simulink model "project2old"  (R2012b)
settings: Solver=ode3  StartTime=0.0  StopTime=2  FixedStep=0.01  RelTol=1e-3
values from neighbouring files (symbols this model uses):
  a1 = 500    [RRR_LinkParameters.m]
  a1s = a1*0.001    (= 0.5)    [RRR_LinkParameters.m]
  a2 = 260    [RRR_LinkParameters.m]
  a2s = a2*0.001    (= 0.26)    [RRR_LinkParameters.m]
  a3 = 50    [RRR_LinkParameters.m]
  g = 9.81    [RRR_LinkParameters.m]
  I1 = 0.0123571    [RRR_LinkParameters.m]
  I2 = 0.00189339    [RRR_LinkParameters.m]
  I3 = 0.0000137671    (= 1.37671e-05)    [RRR_LinkParameters.m]
  L1 = 0.246193    [RRR_LinkParameters.m]
  L2 = 0.626297-0.5    (= 0.126297)    [RRR_LinkParameters.m]
  L3 = 0.780098-0.76    (= 0.020098)    [RRR_LinkParameters.m]
  m1 = 0.556965    [RRR_LinkParameters.m]
  m2 = 0.297765    [RRR_LinkParameters.m]
  m3 = 0.0528412    [RRR_LinkParameters.m]
libraries: mblibv1 x23, simulink x8
settings Model: Creator=Sony  LastModifiedBy=Sony
settings SimMechanicsCC: VisDuringSimulation=on
settings ConfigurationSet: Description=SimMechanics 2G

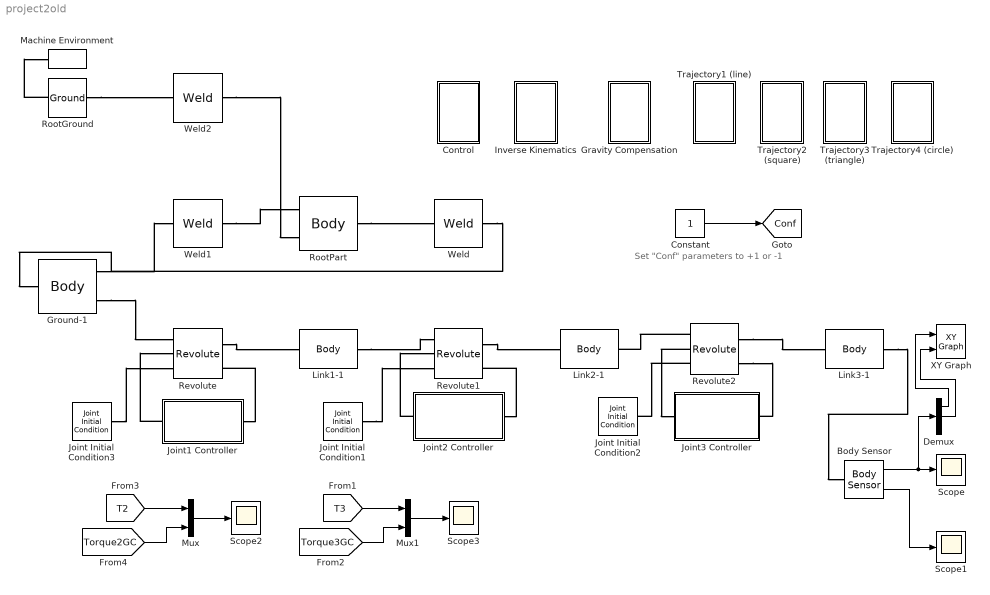
== system project2old ==
  note: Set "Conf" parameters to +1 or -1
  Body Sensor : mblibv1/Sensors &  Actuators/Body Sensor  UpdateFromCAD=off  PhysicalDomain=Mechanical  PortType=blob  Muxed=off  Pose=on  Angle=on  AngleUnits=deg  ArcVelocity=off  ArcVelocityUnits=deg/s  ArcAcceleration=off  ArcAccelerationUnits=deg/s^2  CoordPosition=on  CoordPositionUnits=mm  Velocity=off  VelocityUnits=m/s  Acceleration=off  AccelerationUnits=m/s^2  Quaternion=on  QuaternionDT=off  QuaternionDDT=off  QuaternionUnits=off  OutputVector=[1]  ActiveIO=on  Width=12  DialogClass=MechanicalSensorBlock  ReferenceFrame=Absolute (World)
  Constant : Constant
  Control : Subsystem
  Demux : Demux  Outputs=3
  Gravity Compensation : Subsystem
  Ground-1 : mblibv1/Bodies/Body  LConnTagsString=CS2  RConnTagsString=CS3|CS4  UpdateFromCAD=on  DialogClass=MechanicalBodyBlock  Mass=0.0821588  MassUnits=kg  InertiaUnits=kg*m^2  Inertia=[1.42321e-05,0,0;0,1.42321e-05,0;0,0,2.2987e-05]  Shape=Cylinder  ShapeDims=[1 1]  ShapeUnits=m  ShapeUse=false  Density=1  DensityUnits=kg/m^3  DensityUse=false  GraphicsMode=GFXFILE  GraphicsFileName=Montaj_3R - Ground-1.STL  BodyColorSelMode=COLORPALETTE  BodyColor=[0.894118;0.913725;0.929412]  AttachedToCS=CS1  CG=Right$CG$[0 0 0.01]$WORLD$WORLD$m$[1 0 0;0 1 0;0 0 1]$3x3 Transform$rad$WORLD$false$none  WorkingFrames=Right$CS1$[0 0 0]$WORLD$WORLD$m$[1 0 0;0 1 0;0 0 1]$3x3 Transform$rad$WORLD$false$none#Left$CS2$[0 0 0.01]$WORLD$WORLD$m$[1 0 0;0 1 0;0 0 1]$3x3 Transform$rad$WORLD$true$none#Right$CS3$[0 0 0.01]$WORLD$WORLD$m$[1 0 0;0 1 0;0 0 1]$3x3 Transform$rad$WORLD$true$none#Right$CS4$[0 0 0.02]$WORLD$WORLD$m$[1 0 0;0 1 0;0 0 1]$3x3 Transform$rad$WORLD$true$none  CGPos=[0 0 0.01]  CGRot=[1 0 0;0 1 0;0 0 1]  CS0Pos=[]  CS0Rot=[]  CS1Pos=[0 0 0]  CS1Rot=[1 0 0;0 1 0;0 0 1]  CS2Pos=[0 0 0.01]  CS2Rot=[1 0 0;0 1 0;0 0 1]  CS3Pos=[0 0 0.01]  CS3Rot=[1 0 0;0 1 0;0 0 1]  CS4Pos=[0 0 0.02]  CS4Rot=[1 0 0;0 1 0;0 0 1]  CS5Pos=[]  CS5Rot=[]  CS6Pos=[]  CS6Rot=[]  CS7Pos=[]  CS7Rot=[]  CS8Pos=[]  CS8Rot=[]  CS9Pos=[]  CS9Rot=[]  CS10Pos=[]  CS10Rot=[]  CS11Pos=[]  CS11Rot=[]  CS12Pos=[]  CS12Rot=[]  CS13Pos=[]  CS13Rot=[]  CS14Pos=[]  CS14Rot=[]  CS15Pos=[]  CS15Rot=[]  CS16Pos=[]  CS16Rot=[]  CS17Pos=[]  CS17Rot=[]  CS18Pos=[]  CS18Rot=[]  CS19Pos=[]  CS19Rot=[]  CS20Pos=[]  CS20Rot=[]
  Inverse Kinematics : Subsystem
  Joint Initial Condition1 : mblibv1/Sensors &  Actuators/Joint Initial Condition  UpdateFromCAD=off  LeftPortType=blob  RightPortType=blob  PhysicalDomain=mechanical  DialogClass=InitialConditionBlock  InitialConditions=P1$false$0$m$deg$0$m/s$deg/s#P2$false$0$m$deg$0$m/s$deg/s#P3$false$0$m$deg$0$m/s$deg/s#R1$true$168.86$m$deg$0$m/s$deg/s#R2$false$0$m$deg$0$m/s$deg/s#R3$false$0$m$deg$0$m/s$deg/s#S$false$0$m$deg$0$m/s$deg/s  P1PIC=0  P1VIC=0  P2PIC=0  P2VIC=0  P3PIC=0  P3VIC=0  R1PIC=168.86  R1VIC=0  R2PIC=0  R2VIC=0  R3PIC=0  R3VIC=0  SPIC=0  SVIC=0
  Joint Initial Condition2 : mblibv1/Sensors &  Actuators/Joint Initial Condition  UpdateFromCAD=off  LeftPortType=blob  RightPortType=blob  PhysicalDomain=mechanical  DialogClass=InitialConditionBlock  InitialConditions=P1$false$0$m$deg$0$m/s$deg/s#P2$false$0$m$deg$0$m/s$deg/s#P3$false$0$m$deg$0$m/s$deg/s#R1$true$-104.13$m$deg$0$m/s$deg/s#R2$false$0$m$deg$0$m/s$deg/s#R3$false$0$m$deg$0$m/s$deg/s#S$false$0$m$deg$0$m/s$deg/s  P1PIC=0  P1VIC=0  P2PIC=0  P2VIC=0  P3PIC=0  P3VIC=0  R1PIC=-104.13  R1VIC=0  R2PIC=0  R2VIC=0  R3PIC=0  R3VIC=0  SPIC=0  SVIC=0
  Joint Initial Condition3 : mblibv1/Sensors &  Actuators/Joint Initial Condition  UpdateFromCAD=off  LeftPortType=blob  RightPortType=blob  PhysicalDomain=mechanical  DialogClass=InitialConditionBlock  InitialConditions=P1$false$0$m$deg$0$m/s$deg/s#P2$false$0$m$deg$0$m/s$deg/s#P3$false$0$m$deg$0$m/s$deg/s#R1$true$25.27$m$deg$0$m/s$deg/s#R2$false$0$m$deg$0$m/s$deg/s#R3$false$0$m$deg$0$m/s$deg/s#S$false$0$m$deg$0$m/s$deg/s  P1PIC=0  P1VIC=0  P2PIC=0  P2VIC=0  P3PIC=0  P3VIC=0  R1PIC=25.27  R1VIC=0  R2PIC=0  R2VIC=0  R3PIC=0  R3VIC=0  SPIC=0  SVIC=0
  Joint1 Controller : Subsystem
  Joint2 Controller : Subsystem
  Joint3 Controller : Subsystem
  Link1-1 : mblibv1/Bodies/Body  LConnTagsString=CS2  RConnTagsString=CS3  UpdateFromCAD=on  DialogClass=MechanicalBodyBlock  Mass=0.556965  MassUnits=kg  InertiaUnits=kg*m^2  Inertia=[3.86731e-05,0,-2.08828e-05;0,0.0123589,0;-2.08828e-05,0,0.0123571]  Shape=Cylinder  ShapeDims=[1 1]  ShapeUnits=m  ShapeUse=false  Density=1  DensityUnits=kg/m^3  DensityUse=false  GraphicsMode=GFXFILE  GraphicsFileName=Montaj_3R - Link1-1.STL  BodyColorSelMode=COLORPALETTE  BodyColor=[0.89412 0.91373 0.92941]  AttachedToCS=CS1  CG=Right$CG$[0.246193 0 -0.0098477]$WORLD$WORLD$m$[-1 0 0;0 -1 0;0 0 1]$3x3 Transform$rad$WORLD$false$none  WorkingFrames=Right$CS1$[0.25 0 -0.02]$WORLD$WORLD$m$[-1 0 0;0 -1 0;0 0 1]$3x3 Transform$rad$WORLD$false$none#Left$CS2$[0 0 0.02]$WORLD$WORLD$m$[1 0 0;0 1 0;0 0 1]$3x3 Transform$rad$WORLD$true$none#Right$CS3$[0.5 0 0]$WORLD$WORLD$m$[1 0 0;0 1 0;0 0 1]$3x3 Transform$rad$WORLD$true$none  CGPos=[0.246193 0 -0.0098477]  CGRot=[-1 0 0;0 -1 0;0 0 1]  CS0Pos=[]  CS0Rot=[]  CS1Pos=[0.25 0 -0.02]  CS1Rot=[-1 0 0;0 -1 0;0 0 1]  CS2Pos=[0 0 0.02]  CS2Rot=[1 0 0;0 1 0;0 0 1]  CS3Pos=[0.5 0 0]  CS3Rot=[1 0 0;0 1 0;0 0 1]  CS4Pos=[]  CS4Rot=[]  CS5Pos=[]  CS5Rot=[]  CS6Pos=[]  CS6Rot=[]  CS7Pos=[]  CS7Rot=[]  CS8Pos=[]  CS8Rot=[]  CS9Pos=[]  CS9Rot=[]  CS10Pos=[]  CS10Rot=[]  CS11Pos=[]  CS11Rot=[]  CS12Pos=[]  CS12Rot=[]  CS13Pos=[]  CS13Rot=[]  CS14Pos=[]  CS14Rot=[]  CS15Pos=[]  CS15Rot=[]  CS16Pos=[]  CS16Rot=[]  CS17Pos=[]  CS17Rot=[]  CS18Pos=[]  CS18Rot=[]  CS19Pos=[]  CS19Rot=[]  CS20Pos=[]  CS20Rot=[]
  Link2-1 : mblibv1/Bodies/Body  LConnTagsString=CS2  RConnTagsString=CS3  UpdateFromCAD=on  DialogClass=MechanicalBodyBlock  Mass=0.297765  MassUnits=kg  InertiaUnits=kg*m^2  Inertia=[2.13819e-05,0,-1.07129e-05;0,0.0018952,0;-1.07129e-05,0,0.00189339]  Shape=Cylinder  ShapeDims=[1 1]  ShapeUnits=m  ShapeUse=false  Density=1  DensityUnits=kg/m^3  DensityUse=false  GraphicsMode=GFXFILE  GraphicsFileName=Montaj_3R - Link2-1.STL  BodyColorSelMode=COLORPALETTE  BodyColor=[0.89412 0.91373 0.92941]  AttachedToCS=CS1  CG=Right$CG$[0.626297 0 -0.0297151]$WORLD$WORLD$m$[-1 0 0;0 -1 0;0 0 1]$3x3 Transform$rad$WORLD$false$none  WorkingFrames=Right$CS1$[0.63 0 -0.04]$WORLD$WORLD$m$[-1 0 0;0 -1 0;0 0 1]$3x3 Transform$rad$WORLD$false$none#Left$CS2$[0.5 0 0]$WORLD$WORLD$m$[1 0 0;0 1 0;0 0 1]$3x3 Transform$rad$WORLD$true$none#Right$CS3$[0.76 0 -0.04]$WORLD$WORLD$m$[1 0 0;0 1 0;0 0 1]$3x3 Transform$rad$WORLD$true$none  CGPos=[0.626297 0 -0.0297151]  CGRot=[-1 0 0;0 -1 0;0 0 1]  CS0Pos=[]  CS0Rot=[]  CS1Pos=[0.63 0 -0.04]  CS1Rot=[-1 0 0;0 -1 0;0 0 1]  CS2Pos=[0.5 0 0]  CS2Rot=[1 0 0;0 1 0;0 0 1]  CS3Pos=[0.76 0 -0.04]  CS3Rot=[1 0 0;0 1 0;0 0 1]  CS4Pos=[]  CS4Rot=[]  CS5Pos=[]  CS5Rot=[]  CS6Pos=[]  CS6Rot=[]  CS7Pos=[]  CS7Rot=[]  CS8Pos=[]  CS8Rot=[]  CS9Pos=[]  CS9Rot=[]  CS10Pos=[]  CS10Rot=[]  CS11Pos=[]  CS11Rot=[]  CS12Pos=[]  CS12Rot=[]  CS13Pos=[]  CS13Rot=[]  CS14Pos=[]  CS14Rot=[]  CS15Pos=[]  CS15Rot=[]  CS16Pos=[]  CS16Rot=[]  CS17Pos=[]  CS17Rot=[]  CS18Pos=[]  CS18Rot=[]  CS19Pos=[]  CS19Rot=[]  CS20Pos=[]  CS20Rot=[]
  Link3-1 : mblibv1/Bodies/Body  LConnTagsString=CS2  RConnTagsString=CS1  UpdateFromCAD=on  DialogClass=MechanicalBodyBlock  Mass=0.0528412  MassUnits=kg  InertiaUnits=kg*m^2  Inertia=[3.47692e-06,0,0;0,1.38129e-05,0;0,0,1.37671e-05]  Shape=Cylinder  ShapeDims=[1 1]  ShapeUnits=m  ShapeUse=false  Density=1  DensityUnits=kg/m^3  DensityUse=false  GraphicsMode=GFXFILE  GraphicsFileName=Montaj_3R - Link3-1.STL  BodyColorSelMode=COLORPALETTE  BodyColor=[0.89412 0.91373 0.92941]  AttachedToCS=CS1  CG=Right$CG$[0.780098 0 -0.05]$WORLD$WORLD$m$[1 0 0;0 1 0;0 0 1]$3x3 Transform$rad$WORLD$false$none  WorkingFrames=Right$CS3$[a3 0 0]$Adjoining$Adjoining$mm$[1 0 0;0 1 0;0 0 1]$3x3 Transform$rad$WORLD$false$none#Right$CS1$[0.81 0 -0.06]$WORLD$WORLD$m$[1 0 0;0 1 0;0 0 1]$3x3 Transform$rad$WORLD$true$none#Left$CS2$[0.76 0 -0.04]$WORLD$WORLD$m$[1 0 0;0 1 0;0 0 1]$3x3 Transform$rad$WORLD$true$none  CGPos=[0.780098 0 -0.05]  CGRot=[1 0 0;0 1 0;0 0 1]  CS0Pos=[]  CS0Rot=[]  CS1Pos=[0.81 0 -0.06]  CS1Rot=[1 0 0;0 1 0;0 0 1]  CS2Pos=[0.76 0 -0.04]  CS2Rot=[1 0 0;0 1 0;0 0 1]  CS3Pos=[a3 0 0]  CS3Rot=[1 0 0;0 1 0;0 0 1]  CS4Pos=[]  CS4Rot=[]  CS5Pos=[]  CS5Rot=[]  CS6Pos=[]  CS6Rot=[]  CS7Pos=[]  CS7Rot=[]  CS8Pos=[]  CS8Rot=[]  CS9Pos=[]  CS9Rot=[]  CS10Pos=[]  CS10Rot=[]  CS11Pos=[]  CS11Rot=[]  CS12Pos=[]  CS12Rot=[]  CS13Pos=[]  CS13Rot=[]  CS14Pos=[]  CS14Rot=[]  CS15Pos=[]  CS15Rot=[]  CS16Pos=[]  CS16Rot=[]  CS17Pos=[]  CS17Rot=[]  CS18Pos=[]  CS18Rot=[]  CS19Pos=[]  CS19Rot=[]  CS20Pos=[]  CS20Rot=[]
  Machine Environment : mblibv1/Bodies/Machine Environment  PortType=env  PhysicalDomain=Mechanical  DialogTemplateClass=MECH.MachineEnvironment  SyncWhenCopied=off  Gravity=[0 -9.81 0]  GravityUnits=m/s^2  GravityAsSignal=off  Dimensionality=Auto-detect  AnalysisType=Forward dynamics  LinearAssemblyTolerance=1e-3  LinearAssemblyToleranceUnits=m  AngularAssemblyTolerance=1e-3  AngularAssemblyToleranceUnits=rad  ConstraintSolverType=Stabilizing  ConstraintRelTolerance=1e-4  ConstraintAbsTolerance=1e-4  UseRobustSingularityHandling=off  RedundancyAnalysisToleranceType=Automatically select tolerance  RedundancyAnalysisTolerance=1e-14  StatePerturbationType=Fixed  PerturbationSize=1e-5  VisualizeMachine=on  BodyVisualizationType=Use model default body geometries  BodyColorSelMode=Use model default  DefaultBodyColor=[1 0 0]
  Mux : Mux  Inputs=2
  Mux1 : Mux  Inputs=2
  Revolute : mblibv1/Joints/Revolute  LConnTagsString=__newl0|SA1|SA2  RConnTagsString=__newr0|SA1  UpdateFromCAD=on  NumSAPorts=3  CutJoint=off  MarkAsCut=off  Primitives=prismatic  PrimitiveProps=R1$World$[0,0,1]$revolute  DialogClass=JointBlock  R1Axis=[0,0,1]
  Revolute1 : mblibv1/Joints/Revolute  LConnTagsString=__newl0|SA1|SA2  RConnTagsString=__newr0|SA1  UpdateFromCAD=on  NumSAPorts=3  CutJoint=off  MarkAsCut=off  Primitives=prismatic  PrimitiveProps=R1$World$[0,0,1]$revolute  DialogClass=JointBlock  R1Axis=[0,0,1]
  Revolute2 : mblibv1/Joints/Revolute  LConnTagsString=__newl0|SA1|SA2  RConnTagsString=__newr0|SA1  UpdateFromCAD=on  NumSAPorts=3  CutJoint=off  MarkAsCut=off  Primitives=prismatic  PrimitiveProps=R1$World$[0,0,1]$revolute  DialogClass=JointBlock  R1Axis=[0,0,1]
  RootGround : mblibv1/Bodies/Ground  UpdateFromCAD=on  LeftPortType=env  RightPortType=workingframe  PhysicalDomain=Mechanical  DialogClass=GroundBlock  CoordPosition=[0.368617,0,-0.016321]  CoordPositionUnits=m  StateVectorMgrId=0  MachineId=[1 0]  ShowEnvPort=on
  RootPart : mblibv1/Bodies/Body  LConnTagsString=CS3|CS4  RConnTagsString=CS2  UpdateFromCAD=on  DialogClass=MechanicalBodyBlock  Mass=0  MassUnits=kg  InertiaUnits=kg*m^2  Inertia=[0,0,0;0,0,0;0,0,0]  Shape=Cylinder  ShapeDims=[1 1]  ShapeUnits=m  ShapeUse=false  Density=1  DensityUnits=kg/m^3  DensityUse=false  GraphicsMode=MACHINE_DEFAULT  BodyColorSelMode=MACHINE_DEFAULT  BodyColor=[1;0;0]  AttachedToCS=CS1  CG=Right$CG$[0.368617 0 -0.016321]$WORLD$WORLD$m$[1 0 0;0 1 0;0 0 1]$3x3 Transform$rad$WORLD$false$none  WorkingFrames=Right$CS1$[0 0 0]$WORLD$WORLD$m$[1 0 0;0 1 0;0 0 1]$3x3 Transform$rad$WORLD$false$none#Right$CS2$[0 0 0.01]$WORLD$WORLD$m$[1 0 0;0 1 0;0 0 1]$3x3 Transform$rad$WORLD$true$none#Left$CS3$[0 0 0.01]$WORLD$WORLD$m$[1 0 0;0 1 0;0 0 1]$3x3 Transform$rad$WORLD$true$none#Left$CS4$[0.368617 0 -0.016321]$WORLD$WORLD$m$[1 0 0;0 1 0;0 0 1]$3x3 Transform$rad$WORLD$true$none  CGPos=[0.368617 0 -0.016321]  CGRot=[1 0 0;0 1 0;0 0 1]  CS0Pos=[]  CS0Rot=[]  CS1Pos=[0 0 0]  CS1Rot=[1 0 0;0 1 0;0 0 1]  CS2Pos=[0 0 0.01]  CS2Rot=[1 0 0;0 1 0;0 0 1]  CS3Pos=[0 0 0.01]  CS3Rot=[1 0 0;0 1 0;0 0 1]  CS4Pos=[0.368617 0 -0.016321]  CS4Rot=[1 0 0;0 1 0;0 0 1]  CS5Pos=[]  CS5Rot=[]  CS6Pos=[]  CS6Rot=[]  CS7Pos=[]  CS7Rot=[]  CS8Pos=[]  CS8Rot=[]  CS9Pos=[]  CS9Rot=[]  CS10Pos=[]  CS10Rot=[]  CS11Pos=[]  CS11Rot=[]  CS12Pos=[]  CS12Rot=[]  CS13Pos=[]  CS13Rot=[]  CS14Pos=[]  CS14Rot=[]  CS15Pos=[]  CS15Rot=[]  CS16Pos=[]  CS16Rot=[]  CS17Pos=[]  CS17Rot=[]  CS18Pos=[]  CS18Rot=[]  CS19Pos=[]  CS19Rot=[]  CS20Pos=[]  CS20Rot=[]
  Scope{,1..3} (4 alike) : Scope
      Scope2 settings: YMin=-0.51  YMax=-0.28  SaveName=ScopeData4
      Scope3 settings: TimeRange=2  YMin=-0.011  YMax=0.002  SaveName=ScopeData5
  Trajectory1 (line) : Subsystem
  Trajectory2 (square) : Subsystem
  Trajectory3 (triangle) : Subsystem
  Trajectory4 (circle) : Subsystem
  Weld : mblibv1/Joints/Weld  LConnTagsString=__newl0  RConnTagsString=__newr0  UpdateFromCAD=on  NumSAPorts=0  CutJoint=off  MarkAsCut=off  Primitives=weld  PrimitiveProps=W$WORLD$[0.57735,0.57735,0.57735]$weld  DialogClass=JointBlock  WAxis=[0.57735,0.57735,0.57735]
  Weld1 : mblibv1/Joints/Weld  LConnTagsString=__newl0  RConnTagsString=__newr0  UpdateFromCAD=on  NumSAPorts=0  CutJoint=off  MarkAsCut=off  Primitives=weld  PrimitiveProps=W$WORLD$[0.57735,0.57735,0.57735]$weld  DialogClass=JointBlock  WAxis=[0.57735,0.57735,0.57735]
  Weld2 : mblibv1/Joints/Weld  LConnTagsString=__newl0  RConnTagsString=__newr0  UpdateFromCAD=on  NumSAPorts=0  CutJoint=off  MarkAsCut=off  Primitives=weld  PrimitiveProps=W$WORLD$[0.57735,0.57735,0.57735]$weld  DialogClass=JointBlock  WAxis=[0.57735,0.57735,0.57735]
  XY Graph : simulink/Sinks/XY Graph  xmin=150  xmax=400  ymin=100  ymax=300  st=-1
  tag scope: Conf=global
  wires:
  Body Sensor/1 -> Demux/1, Scope/1
  Body Sensor/2 -> Scope1/1
  Constant/1 -> [Conf]
  Demux/1 -> XY Graph/1
  Demux/2 -> XY Graph/2
  Mux/1 -> Scope2/1
  [T2] -> Mux/1
  [Torque2GC] -> Mux/2
  Mux1/1 -> Scope3/1
  [T3] -> Mux1/1
  [Torque3GC] -> Mux1/2
  connections:
  Revolute1/RConn1 -- Link2-1/LConn1
  Revolute2/LConn1 -- Link2-1/RConn1
  Link1-1/RConn1 -- Revolute1/LConn1
  Link3-1/RConn1 -- Body Sensor/LConn1
  Ground-1/RConn1 -- Weld1/LConn1
  Revolute2/RConn1 -- Link3-1/LConn1
  Weld1/RConn1 -- RootPart/LConn1
  Weld2/RConn1 -- RootPart/LConn2
  Weld/RConn1 -- Ground-1/LConn1
  RootGround/RConn1 -- Weld2/LConn1
  Revolute/RConn1 -- Link1-1/LConn1
  Ground-1/RConn2 -- Revolute/LConn1
  RootPart/RConn1 -- Weld/LConn1
  RootGround/LConn1 -- Machine Environment/RConn1
  Joint2 Controller/LConn1 -- Revolute1/LConn2
  Joint2 Controller/RConn1 -- Revolute1/RConn2
  Revolute2/LConn2 -- Joint3 Controller/LConn1
  Revolute2/RConn2 -- Joint3 Controller/RConn1
  Joint1 Controller/RConn1 -- Revolute/LConn2
  Joint1 Controller/LConn1 -- Revolute/RConn2
  Joint Initial Condition3/RConn1 -- Revolute/LConn3
  Joint Initial Condition1/RConn1 -- Revolute1/LConn3
  Revolute2/LConn3 -- Joint Initial Condition2/RConn1

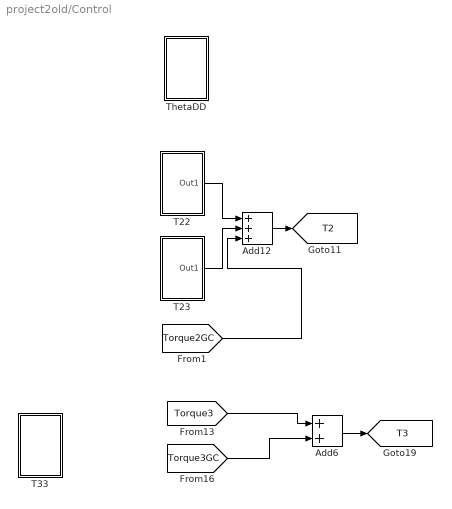
== system project2old/Control ==
  Add12 : Sum  Inputs=+++
  Add6 : Sum
  T22 : Subsystem
  T23 : Subsystem
  T33 : Subsystem
  ThetaDD : Subsystem
  tag scope: T2=global, T3=global
  wires:
  [Torque3] -> Add6/1
  [Torque3GC] -> Add6/2
  Add6/1 -> [T3]
  T22/1(Out1) -> Add12/1
  T23/1(Out1) -> Add12/2
  Add12/1 -> [T2]
  [Torque2GC] -> Add12/3

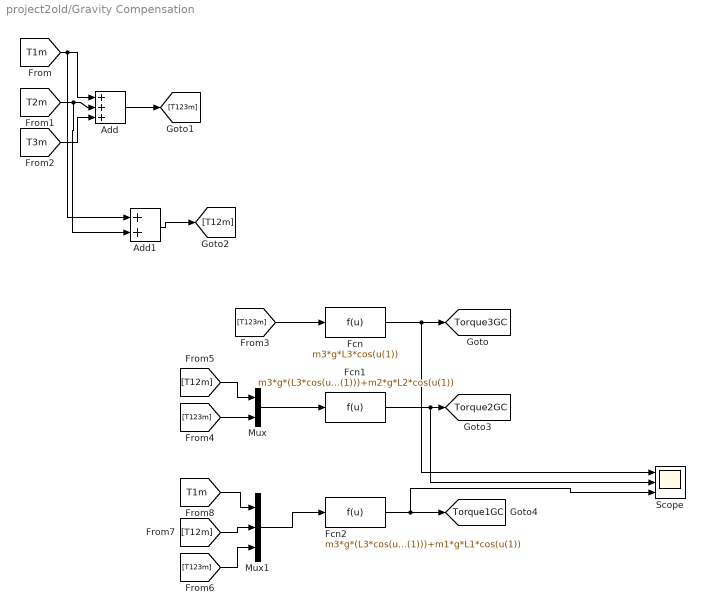
== system project2old/Gravity Compensation ==
  Add : Sum  Inputs=+++
  Add1 : Sum
  Fcn : Fcn  Expr=m3*g*L3*cos(u(1))
  Fcn1 : Fcn  Expr=m3*g*(L3*cos(u(2))+a2s*cos(u(1)))+m2*g*L2*cos(u(1))
  Fcn2 : Fcn  Expr=m3*g*(L3*cos(u(3))+a2s*cos(u(2))+a1s*cos(u(1)))+m2*g*(L2*cos(u(2))+a1s*cos(u(1)))+m1*g*L1*cos(u(1))
  Mux : Mux  Inputs=2
  Mux1 : Mux  Inputs=3
  Scope : Scope  NumInputPorts=3
      settings: YMin=-5~-5~-5  YMax=5~5~5
  tag scope: Torque1GC=global, Torque2GC=global, Torque3GC=global
  wires:
  [T3m] -> Add/3
  [T1m] -> Add1/1, Add/1
  [T2m] -> Add1/2, Add/2
  Add/1 -> [T123m]
  Add1/1 -> [T12m]
  [T123m] -> Fcn/1
  Fcn/1 -> Scope/1, [Torque3GC]
  Fcn1/1 -> Scope/2, [Torque2GC]
  [T12m] -> Mux/1
  [T123m] -> Mux/2
  Mux/1 -> Fcn1/1
  Fcn2/1 -> Scope/3, [Torque1GC]
  Mux1/1 -> Fcn2/1
  [T1m] -> Mux1/1
  [T12m] -> Mux1/2
  [T123m] -> Mux1/3

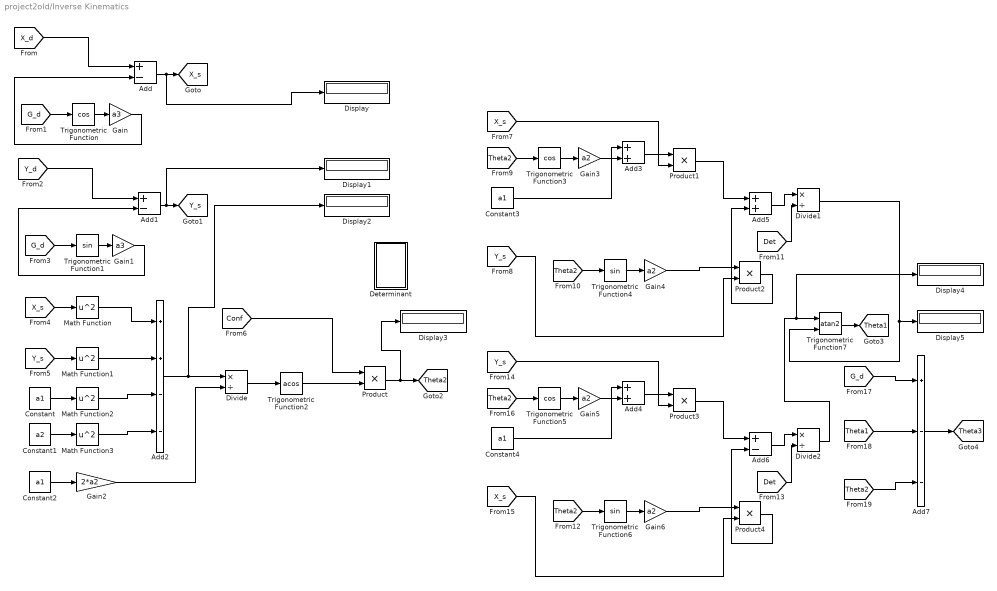
== system project2old/Inverse Kinematics ==
  Add : Sum  Inputs=+-
  Add1 : Sum  Inputs=+-
  Add2 : Sum  Inputs=++--
  Add3 : Sum
  Add4 : Sum
  Add5 : Sum
  Add6 : Sum  Inputs=+-
  Add7 : Sum  Inputs=+--
  Constant{,2..4} (4 alike) : Constant  Value=a1
  Constant1 : Constant  Value=a2
  Determinant : Subsystem
  Display{,1..5} (6 alike) : Display
  Divide : Product  Inputs=*/
  Divide1 : Product  Inputs=*/
  Divide2 : Product  Inputs=*/
  Gain : Gain  Gain=a3
  Gain1 : Gain  Gain=a3
  Gain2 : Gain  Gain=2*a2
  Gain{3..6} (4 alike) : Gain  Gain=a2
  Math Function{,1..3} (4 alike) : Math  Operator=square  SaturateOnIntegerOverflow=on
  Product{,1..4} (5 alike) : Product  RndMeth=Zero
  Trigonometric Function : Trigonometry  Operator=cos
  Trigonometric Function1 : Trigonometry
  Trigonometric Function2 : Trigonometry  Operator=acos
  Trigonometric Function3 : Trigonometry  Operator=cos
  Trigonometric Function4 : Trigonometry
  Trigonometric Function5 : Trigonometry  Operator=cos
  Trigonometric Function6 : Trigonometry
  Trigonometric Function7 : Trigonometry  Operator=atan2
  tag scope: Theta1=global, Theta2=global, Theta3=global, X_s=global, Y_s=global
  wires:
  Add1/1 -> Display1/1, [Y_s]
  [X_d] -> Add/1
  Add/1 -> Display/1, [X_s]
  [Y_d] -> Add1/1
  Gain/1 -> Add/2
  [G_d] -> Trigonometric Function1/1
  Trigonometric Function/1 -> Gain/1
  [G_d] -> Trigonometric Function/1
  Gain1/1 -> Add1/2
  Trigonometric Function1/1 -> Gain1/1
  [X_s] -> Math Function/1
  [Y_s] -> Math Function1/1
  Constant1/1 -> Math Function3/1
  Constant/1 -> Math Function2/1
  Math Function3/1 -> Add2/4
  Math Function2/1 -> Add2/3
  Math Function1/1 -> Add2/2
  Math Function/1 -> Add2/1
  Add2/1 -> Display2/1, Divide/1
  Constant2/1 -> Gain2/1
  Gain2/1 -> Divide/2
  Divide/1 -> Trigonometric Function2/1
  Trigonometric Function2/1 -> Product/2
  [Conf] -> Product/1
  Product/1 -> Display3/1, [Theta2]
  [Theta2] -> Trigonometric Function3/1
  Trigonometric Function3/1 -> Gain3/1
  Gain3/1 -> Add3/2
  Constant3/1 -> Add3/1
  Add3/1 -> Product1/1
  [X_s] -> Product1/2
  [Theta2] -> Trigonometric Function4/1
  Trigonometric Function4/1 -> Gain4/1
  [Y_s] -> Product2/2
  Product2/1 -> Add5/2
  Gain4/1 -> Product2/1
  Add5/1 -> Divide1/1
  [Det] -> Divide1/2
  Product1/1 -> Add5/1
  [Theta2] -> Trigonometric Function5/1
  Trigonometric Function5/1 -> Gain5/1
  Gain5/1 -> Add4/2
  Constant4/1 -> Add4/1
  Add4/1 -> Product3/1
  [Y_s] -> Product3/2
  [Theta2] -> Trigonometric Function6/1
  Trigonometric Function6/1 -> Gain6/1
  [X_s] -> Product4/2
  Product4/1 -> Add6/2
  Gain6/1 -> Product4/1
  Add6/1 -> Divide2/1
  [Det] -> Divide2/2
  Product3/1 -> Add6/1
  Trigonometric Function7/1 -> [Theta1]
  [Theta2] -> Add7/3
  [Theta1] -> Add7/2
  [G_d] -> Add7/1
  Add7/1 -> [Theta3]
  Divide2/1 -> Display4/1, Trigonometric Function7/1
  Divide1/1 -> Display5/1, Trigonometric Function7/2

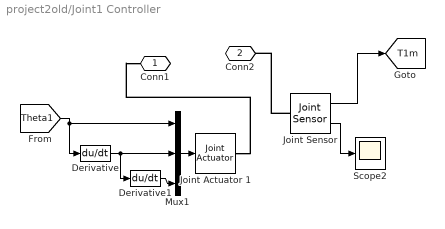
== system project2old/Joint1 Controller ==
  Derivative : Derivative
  Derivative1 : Derivative
  Joint Actuator 1 : mblibv1/Sensors &  Actuators/Joint Actuator  UpdateFromCAD=off  PhysicalDomain=Mechanical  PortType=blob  ActuationStyle=Motion  AngleUnits=rad  ArcVelocityUnits=rad/s  ArcAccelerationUnits=rad/s^2  CoordPositionUnits=m  VelocityUnits=m/s  AccelerationUnits=m/s^2  ForceUnits=N  TorqueUnits=N*m  ActiveIO=on  Width=3  DialogClass=MechanicalActuatorBlock  Primitive=R1  ReferenceFrame=Absolute (World)
  Joint Sensor : mblibv1/Sensors &  Actuators/Joint Sensor  UpdateFromCAD=off  PhysicalDomain=Mechanical  PortType=blob  Muxed=off  Pose=off  Angle=on  AngleUnits=rad  ArcVelocity=off  ArcVelocityUnits=deg/s  ArcAcceleration=off  ArcAccelerationUnits=deg/s^2  CoordPosition=on  CoordPositionUnits=m  Velocity=off  VelocityUnits=m/s  Acceleration=off  AccelerationUnits=m/s^2  Quaternion=on  QuaternionDT=off  QuaternionDDT=off  QuaternionUnits=off  OutputVector=[1]  ActiveIO=on  Width=2  DialogClass=MechanicalSensorBlock  Primitive=R1  Force=off  ForceUnits=N  Torque=on  TorqueUnits=N*m  ReferenceFrame=Absolute (World)  ReactionSensedSide=Base  ReactionReferenceFrame=Absolute (World)  ReactionForce=off  ReactionForceUnits=N  ReactionMoment=off  ReactionMomentUnits=N*m
  Mux1 : Mux  Inputs=3
  Scope2 : Scope
      settings: SaveName=Joint1Torque
  Conn1 : PMIOPort  Port=1  Side=Right
  Conn2 : PMIOPort  Port=2  Side=Left
  tag scope: T1m=global
  wires:
  Mux1/1 -> Joint Actuator 1/1
  Derivative1/1 -> Mux1/3
  Derivative/1 -> Derivative1/1, Mux1/2
  [Theta1] -> Mux1/1, Derivative/1
  Joint Sensor/1 -> [T1m]
  Joint Sensor/2 -> Scope2/1
  connections:
  Joint Sensor/LConn1 -- Conn2/RConn1
  Joint Actuator 1/RConn1 -- Conn1/RConn1

== system project2old/Joint2 Controller ==
  Display : Display
  Joint Actuator : mblibv1/Sensors &  Actuators/Joint Actuator  UpdateFromCAD=off  PhysicalDomain=Mechanical  PortType=blob  ActuationStyle=Force  AngleUnits=deg  ArcVelocityUnits=deg/s  ArcAccelerationUnits=deg/s^2  CoordPositionUnits=m  VelocityUnits=m/s  AccelerationUnits=m/s^2  ForceUnits=N  TorqueUnits=N*m  ActiveIO=on  Width=1  DialogClass=MechanicalActuatorBlock  Primitive=R1  ReferenceFrame=Absolute (World)
  Joint Sensor : mblibv1/Sensors &  Actuators/Joint Sensor  UpdateFromCAD=off  PhysicalDomain=Mechanical  PortType=blob  Muxed=off  Pose=off  Angle=on  AngleUnits=rad  ArcVelocity=off  ArcVelocityUnits=deg/s  ArcAcceleration=off  ArcAccelerationUnits=deg/s^2  CoordPosition=on  CoordPositionUnits=m  Velocity=off  VelocityUnits=m/s  Acceleration=off  AccelerationUnits=m/s^2  Quaternion=on  QuaternionDT=off  QuaternionDDT=off  QuaternionUnits=off  OutputVector=[1]  ActiveIO=on  Width=2  DialogClass=MechanicalSensorBlock  Primitive=R1  Force=off  ForceUnits=N  Torque=on  TorqueUnits=N*m  ReferenceFrame=Absolute (World)  ReactionSensedSide=Base  ReactionReferenceFrame=Absolute (World)  ReactionForce=off  ReactionForceUnits=N  ReactionMoment=off  ReactionMomentUnits=N*m
  Scope2 : Scope
      settings: SaveName=ScopeData3
  Conn1 : PMIOPort  Port=1  Side=Left
  Conn2 : PMIOPort  Port=2  Side=Right
  tag scope: T2m=global
  wires:
  Joint Sensor/1 -> Scope2/1, [T2m]
  Joint Sensor/2 -> Display/1
  [T2] -> Joint Actuator/1
  connections:
  Joint Sensor/LConn1 -- Conn2/RConn1
  Joint Actuator/RConn1 -- Conn1/RConn1

== system project2old/Joint3 Controller ==
  Display : Display
  Joint Actuator : mblibv1/Sensors &  Actuators/Joint Actuator  UpdateFromCAD=off  PhysicalDomain=Mechanical  PortType=blob  ActuationStyle=Force  AngleUnits=rad  ArcVelocityUnits=rad/s  ArcAccelerationUnits=rad/s^2  CoordPositionUnits=m  VelocityUnits=m/s  AccelerationUnits=m/s^2  ForceUnits=N  TorqueUnits=N*m  ActiveIO=on  Width=1  DialogClass=MechanicalActuatorBlock  Primitive=R1  ReferenceFrame=Absolute (World)
  Joint Sensor : mblibv1/Sensors &  Actuators/Joint Sensor  UpdateFromCAD=off  PhysicalDomain=Mechanical  PortType=blob  Muxed=off  Pose=off  Angle=on  AngleUnits=rad  ArcVelocity=off  ArcVelocityUnits=deg/s  ArcAcceleration=off  ArcAccelerationUnits=deg/s^2  CoordPosition=on  CoordPositionUnits=m  Velocity=off  VelocityUnits=m/s  Acceleration=off  AccelerationUnits=m/s^2  Quaternion=on  QuaternionDT=off  QuaternionDDT=off  QuaternionUnits=off  OutputVector=[1]  ActiveIO=on  Width=2  DialogClass=MechanicalSensorBlock  Primitive=R1  Force=off  ForceUnits=N  Torque=on  TorqueUnits=N*m  ReferenceFrame=Absolute (World)  ReactionSensedSide=Base  ReactionReferenceFrame=Absolute (World)  ReactionForce=off  ReactionForceUnits=N  ReactionMoment=off  ReactionMomentUnits=N*m
  Scope2 : Scope
      settings: SaveName=ScopeData2
  Conn1 : PMIOPort  Port=1  Side=Left
  Conn2 : PMIOPort  Port=2  Side=Right
  tag scope: T3m=global
  wires:
  Joint Sensor/1 -> Scope2/1, [T3m]
  [T3] -> Joint Actuator/1
  Joint Sensor/2 -> Display/1
  connections:
  Conn1/RConn1 -- Joint Actuator/RConn1
  Joint Sensor/LConn1 -- Conn2/RConn1

== system project2old/Trajectory1 (line) ==
  Add : Sum
  Constant1 : Constant  Value=pi/2
  Constant2 : Constant  Value=200
  Constant4 : Constant  Value=200
  Integrator : Integrator
  Repeating Sequence : simulink/Sources/Repeating Sequence  rep_seq_t=[0 1 2]  rep_seq_y=[0 100 0]
  tag scope: G_d=global, X_d=global, Y_d=global
  wires:
  Constant4/1 -> Add/1
  Repeating Sequence/1 -> Integrator/1
  Integrator/1 -> Add/2
  Constant2/1 -> [Y_d]
  Add/1 -> [X_d]
  Constant1/1 -> [G_d]

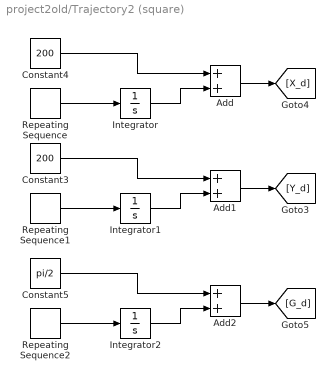
== system project2old/Trajectory2 (square) ==
  Add : Sum
  Add1 : Sum
  Add2 : Sum
  Constant3 : Constant  Value=200
  Constant4 : Constant  Value=200
  Constant5 : Constant  Value=pi/2
  Integrator : Integrator
  Integrator1 : Integrator
  Integrator2 : Integrator
  Repeating Sequence : simulink/Sources/Repeating Sequence  rep_seq_t=[0 1 2 3 4 5 6 7 8 9 10 11 12 13 14]  rep_seq_y=[0 100 0 0 0 0 0 0 0 -100 0 0 0 0 0]
  Repeating Sequence1 : simulink/Sources/Repeating Sequence  rep_seq_t=[0 1 2 3 4 5 6 7 8 9 10 11 12 13 14]  rep_seq_y=[0 0 0 0 0 100 0 0 0 0 0 0 0 -100 0]
  Repeating Sequence2 : simulink/Sources/Repeating Sequence  rep_seq_t=[0 1 2 3 4 5 6 7 8 9 10 11 12 13 14]  rep_seq_y=[0 0 0 pi/2 0 0 0 -pi/2 0 0 0 pi/2 0 0 0]
  wires:
  Add/1 -> [X_d]
  Integrator/1 -> Add/2
  Repeating Sequence/1 -> Integrator/1
  Constant4/1 -> Add/1
  Add1/1 -> [Y_d]
  Integrator1/1 -> Add1/2
  Repeating Sequence1/1 -> Integrator1/1
  Constant3/1 -> Add1/1
  Add2/1 -> [G_d]
  Integrator2/1 -> Add2/2
  Repeating Sequence2/1 -> Integrator2/1
  Constant5/1 -> Add2/1

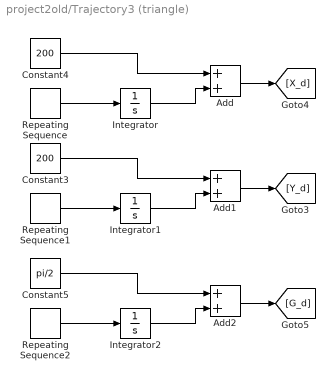
== system project2old/Trajectory3 (triangle) ==
  Add : Sum
  Add1 : Sum
  Add2 : Sum
  Constant3 : Constant  Value=200
  Constant4 : Constant  Value=200
  Constant5 : Constant  Value=pi/2
  Integrator : Integrator
  Integrator1 : Integrator
  Integrator2 : Integrator
  Repeating Sequence : simulink/Sources/Repeating Sequence  rep_seq_t=[0 1 2 3 4 5 6 7 8 9 10]  rep_seq_y=[0 60 0 0 0 -30 0 0 0 -30 0 ]
  Repeating Sequence1 : simulink/Sources/Repeating Sequence  rep_seq_t=[0 1 2 3 4 5 6 7 8 9 10]  rep_seq_y=[0 0 0 0 0 40 0 0 0 -40 0]
  Repeating Sequence2 : simulink/Sources/Repeating Sequence  rep_seq_t=[0 1 2 3 4 5 6 7 8 9 10]  rep_seq_y=[0 0 0 -pi/3.4 0 0 0 pi/2.43 0 0 0]
  wires:
  Add/1 -> [X_d]
  Integrator/1 -> Add/2
  Repeating Sequence/1 -> Integrator/1
  Constant4/1 -> Add/1
  Add1/1 -> [Y_d]
  Integrator1/1 -> Add1/2
  Repeating Sequence1/1 -> Integrator1/1
  Constant3/1 -> Add1/1
  Add2/1 -> [G_d]
  Integrator2/1 -> Add2/2
  Repeating Sequence2/1 -> Integrator2/1
  Constant5/1 -> Add2/1

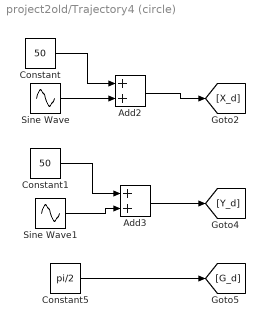
== system project2old/Trajectory4 (circle) ==
  Add2 : Sum
  Add3 : Sum
  Constant : Constant  Value=50
  Constant1 : Constant  Value=50
  Constant5 : Constant  Value=pi/2
  Sine Wave : Sin  Amplitude=20  Frequency=2*pi/100  Phase=pi/2  SampleTime=0
  Sine Wave1 : Sin  Amplitude=20  Frequency=2*pi/100  SampleTime=0
  wires:
  Constant5/1 -> [G_d]
  Constant/1 -> Add2/1
  Sine Wave/1 -> Add2/2
  Constant1/1 -> Add3/1
  Sine Wave1/1 -> Add3/2
  Add2/1 -> [X_d]
  Add3/1 -> [Y_d]

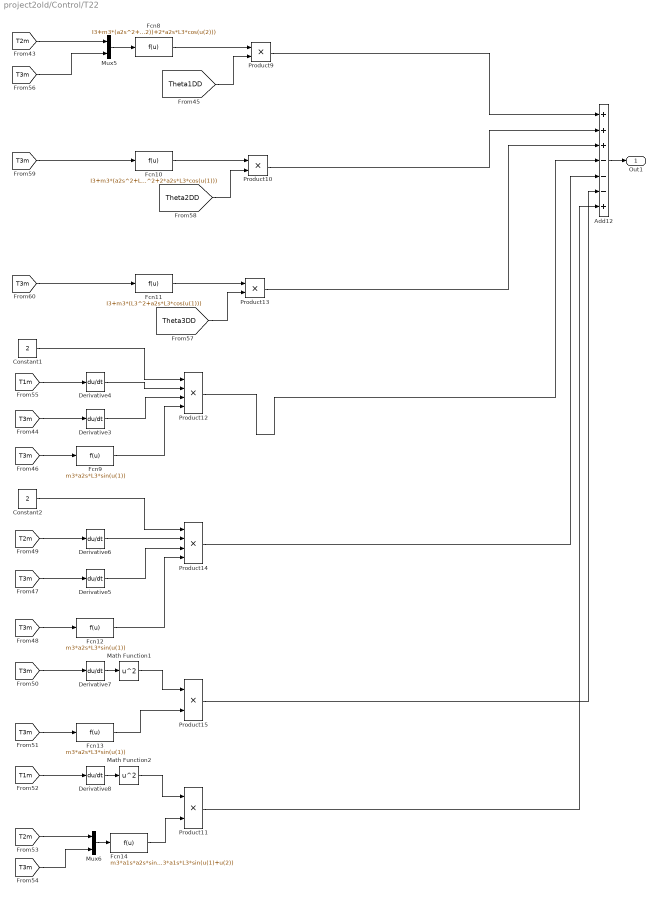
== system project2old/Control/T22 ==
  Add12 : Sum  Inputs=+++---+
  Constant1 : Constant  Value=2
  Constant2 : Constant  Value=2
  Derivative{3..8} (6 alike) : Derivative
  Fcn10 : Fcn  Expr=I3+m3*(a2s^2+L3^2+2*a2s*L3*cos(u(1)))
  Fcn11 : Fcn  Expr=I3+m3*(L3^2+a2s*L3*cos(u(1)))
  Fcn12 : Fcn  Expr=m3*a2s*L3*sin(u(1))
  Fcn13 : Fcn  Expr=m3*a2s*L3*sin(u(1))
  Fcn14 : Fcn  Expr=m3*a1s*a2s*sin(u(1))+m3*a1s*L3*sin(u(1)+u(2))
  Fcn8 : Fcn  Expr=I3+m3*(a2s^2+L3^2+a1s*a2s*cos(u(1))+a1s*L3*cos(u(1)+(2))+2*a2s*L3*cos(u(2)))
  Fcn9 : Fcn  Expr=m3*a2s*L3*sin(u(1))
  Math Function1 : Math  Operator=square  SaturateOnIntegerOverflow=on
  Math Function2 : Math  Operator=square  SaturateOnIntegerOverflow=on
  Mux5 : Mux  Inputs=2
  Mux6 : Mux  Inputs=2
  Product{9..11,13,15} (5 alike) : Product
  Product12 : Product  Inputs=4
  Product14 : Product  Inputs=4
  Out1 : Outport
  wires:
  Add12/1 -> Out1/1
  [T3m] -> Fcn13/1
  [T3m] -> Derivative7/1
  Product10/1 -> Add12/2
  [T3m] -> Fcn10/1
  Fcn9/1 -> Product12/4
  [T1m] -> Derivative4/1
  Math Function2/1 -> Product11/1
  [Theta1DD] -> Product9/2
  [T3m] -> Derivative5/1
  Product11/1 -> Add12/7
  [T3m] -> Fcn12/1
  [Theta2DD] -> Product10/2
  [T3m] -> Fcn9/1
  [T3m] -> Fcn11/1
  Product13/1 -> Add12/3
  Derivative6/1 -> Product14/2
  Product15/1 -> Add12/6
  Product9/1 -> Add12/1
  [T3m] -> Derivative3/1
  Product14/1 -> Add12/5
  [Theta3DD] -> Product13/2
  Derivative8/1 -> Math Function2/1
  [T2m] -> Mux5/1
  Fcn12/1 -> Product14/4
  Constant1/1 -> Product12/1
  Derivative3/1 -> Product12/3
  Derivative7/1 -> Math Function1/1
  Product12/1 -> Add12/4
  [T3m] -> Mux6/2
  Fcn14/1 -> Product11/2
  [T2m] -> Derivative6/1
  Derivative5/1 -> Product14/3
  Fcn11/1 -> Product13/1
  Fcn8/1 -> Product9/1
  Mux6/1 -> Fcn14/1
  Fcn13/1 -> Product15/2
  [T3m] -> Mux5/2
  Mux5/1 -> Fcn8/1
  [T1m] -> Derivative8/1
  Derivative4/1 -> Product12/2
  Fcn10/1 -> Product10/1
  [T2m] -> Mux6/1
  Math Function1/1 -> Product15/1
  Constant2/1 -> Product14/1

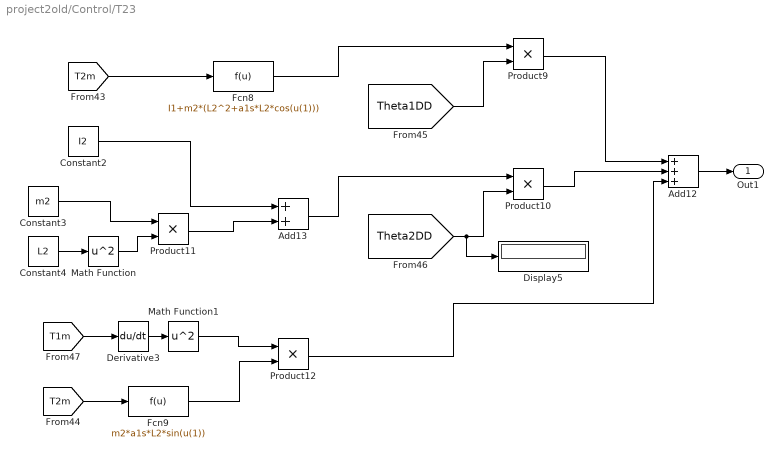
== system project2old/Control/T23 ==
  Add12 : Sum  Inputs=+++
  Add13 : Sum
  Constant2 : Constant  Value=I2
  Constant3 : Constant  Value=m2
  Constant4 : Constant  Value=L2
  Derivative3 : Derivative
  Display5 : Display
  Fcn8 : Fcn  Expr=I1+m2*(L2^2+a1s*L2*cos(u(1)))
  Fcn9 : Fcn  Expr=m2*a1s*L2*sin(u(1))
  Math Function : Math  Operator=square  SaturateOnIntegerOverflow=on
  Math Function1 : Math  Operator=square  SaturateOnIntegerOverflow=on
  Product{9..12} (4 alike) : Product
  Out1 : Outport
  wires:
  [Theta1DD] -> Product9/2
  Product9/1 -> Add12/1
  Math Function1/1 -> Product12/1
  Constant4/1 -> Math Function/1
  Add12/1 -> Out1/1
  [T2m] -> Fcn9/1
  Product11/1 -> Add13/2
  Constant3/1 -> Product11/1
  Math Function/1 -> Product11/2
  Fcn8/1 -> Product9/1
  Derivative3/1 -> Math Function1/1
  Product12/1 -> Add12/3
  [T1m] -> Derivative3/1
  [T2m] -> Fcn8/1
  Constant2/1 -> Add13/1
  Add13/1 -> Product10/1
  Product10/1 -> Add12/2
  [Theta2DD] -> Display5/1, Product10/2
  Fcn9/1 -> Product12/2

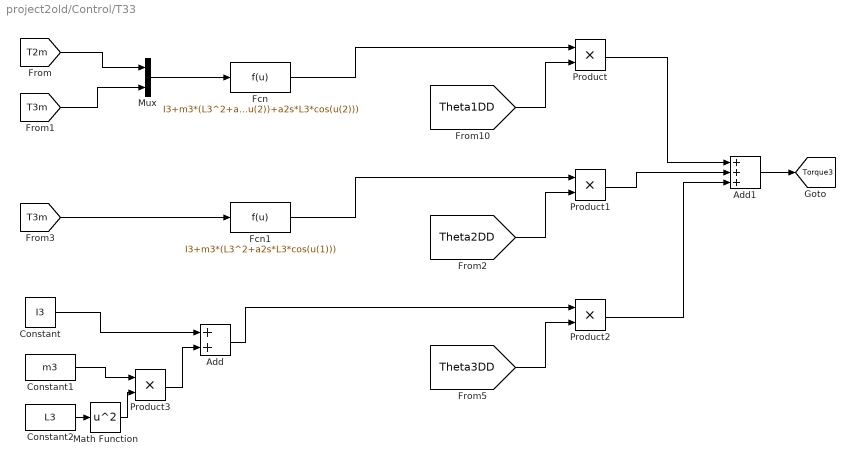
== system project2old/Control/T33 ==
  Add : Sum
  Add1 : Sum  Inputs=+++
  Constant : Constant  Value=I3
  Constant1 : Constant  Value=m3
  Constant2 : Constant  Value=L3
  Fcn : Fcn  Expr=I3+m3*(L3^2+a1s*L3*cos(u(1)+u(2))+a2s*L3*cos(u(2)))
  Fcn1 : Fcn  Expr=I3+m3*(L3^2+a2s*L3*cos(u(1)))
  Math Function : Math  Operator=square  SaturateOnIntegerOverflow=on
  Mux : Mux  Inputs=2
  Product{,1..3} (4 alike) : Product
  tag scope: Torque3=global
  wires:
  Mux/1 -> Fcn/1
  [T3m] -> Fcn1/1
  Constant/1 -> Add/1
  [T2m] -> Mux/1
  [T3m] -> Mux/2
  Fcn1/1 -> Product1/1
  [Theta2DD] -> Product1/2
  Product1/1 -> Add1/2
  Product2/1 -> Add1/3
  Product/1 -> Add1/1
  Fcn/1 -> Product/1
  Add/1 -> Product2/1
  [Theta3DD] -> Product2/2
  [Theta1DD] -> Product/2
  Constant2/1 -> Math Function/1
  Math Function/1 -> Product3/2
  Constant1/1 -> Product3/1
  Product3/1 -> Add/2
  Add1/1 -> [Torque3]

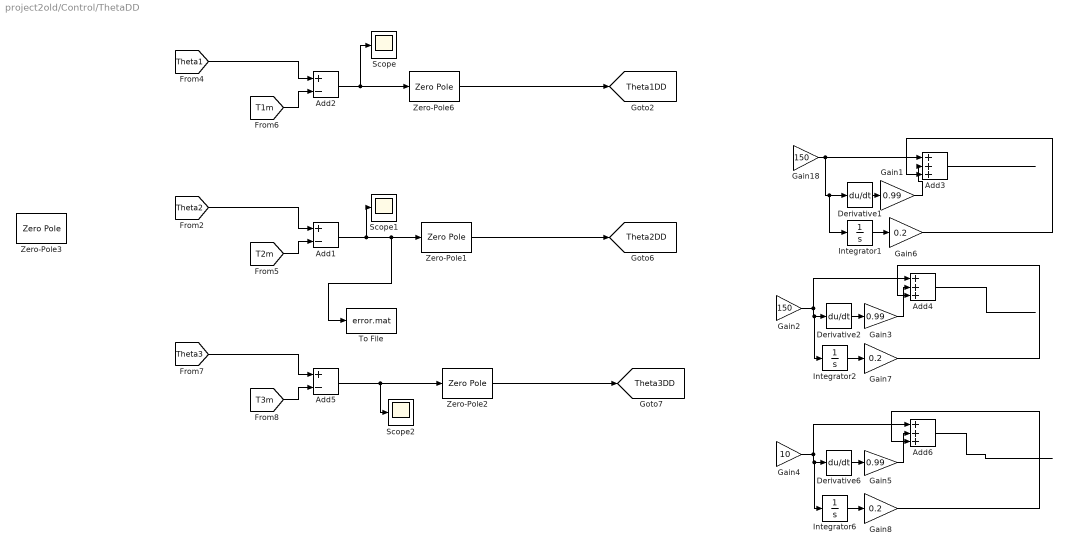
== system project2old/Control/ThetaDD ==
  Add1 : Sum  Inputs=+-
  Add2 : Sum  Inputs=+-
  Add3 : Sum  Inputs=+++
  Add4 : Sum  Inputs=+++
  Add5 : Sum  Inputs=+-
  Add6 : Sum  Inputs=+++
  Derivative1 : Derivative
  Derivative2 : Derivative
  Derivative6 : Derivative
  Gain1 : Gain  Gain=0.99
  Gain18 : Gain  Gain=150
  Gain2 : Gain  Gain=150
  Gain3 : Gain  Gain=0.99
  Gain4 : Gain  Gain=10
  Gain5 : Gain  Gain=0.99
  Gain6 : Gain  Gain=0.2
  Gain7 : Gain  Gain=0.2
  Gain8 : Gain  Gain=0.2
  Integrator1 : Integrator
  Integrator2 : Integrator
  Integrator6 : Integrator
  Scope : Scope
      settings: SaveName=ScopeData7
  Scope1 : Scope
      settings: YMin=-0.09  YMax=0.06  SaveName=ScopeData8
  Scope2 : Scope
      settings: YMin=-1.75  YMax=0.75  SaveName=ScopeData9
  To File : ToFile  Filename=error.mat  MatrixName=error
  Zero-Pole1 : ZeroPole  Zeros=[-10]  Poles=[-20]  Gain=[10000]
  Zero-Pole2 : ZeroPole  Zeros=[-10]  Poles=[-20]  Gain=[10000]
  Zero-Pole3 : ZeroPole  Zeros=[-0.01]  Poles=[-0.009]  Gain=[10000]
  Zero-Pole6 : ZeroPole  Zeros=[-10]  Poles=[-20]  Gain=[10000]
  tag scope: Theta1DD=global, Theta2DD=global, Theta3DD=global
  wires:
  [T2m] -> Add1/2
  [T3m] -> Add5/2
  [T1m] -> Add2/2
  [Theta1] -> Add2/1
  [Theta2] -> Add1/1
  [Theta3] -> Add5/1
  Add5/1 -> Zero-Pole2/1, Scope2/1
  Add1/1 -> Scope1/1, Zero-Pole1/1, To File/1
  Add2/1 -> Zero-Pole6/1, Scope/1
  Derivative1/1 -> Gain1/1
  Gain3/1 -> Add4/2
  Gain18/1 -> Integrator1/1, Derivative1/1, Add3/1
  Gain2/1 -> Add4/1, Integrator2/1, Derivative2/1
  Gain1/1 -> Add3/2
  Derivative2/1 -> Gain3/1
  Derivative6/1 -> Gain5/1
  Gain5/1 -> Add6/2
  Gain4/1 -> Integrator6/1, Derivative6/1, Add6/1
  Integrator6/1 -> Gain8/1
  Gain8/1 -> Add6/3
  Gain7/1 -> Add4/3
  Integrator2/1 -> Gain7/1
  Integrator1/1 -> Gain6/1
  Gain6/1 -> Add3/3
  ? -> Gain4/1
  ? -> Gain2/1
  ? -> Gain18/1
  Add6/1 -> ?
  Add4/1 -> ?
  Add3/1 -> ?
  Zero-Pole1/1 -> [Theta2DD]
  Zero-Pole6/1 -> [Theta1DD]
  Zero-Pole2/1 -> [Theta3DD]

== system project2old/Inverse Kinematics/Determinant ==
  Add4 : Sum  Inputs=+++
  Constant4 : Constant  Value=a1
  Constant5 : Constant  Value=a2
  Gain5 : Gain  Gain=2*a1*a2
  Math Function4 : Math  Operator=square  SaturateOnIntegerOverflow=on
  Math Function5 : Math  Operator=square  SaturateOnIntegerOverflow=on
  Trigonometric Function5 : Trigonometry  Operator=cos
  tag scope: Det=global
  wires:
  Add4/1 -> [Det]
  Math Function4/1 -> Add4/1
  Gain5/1 -> Add4/3
  [Theta2] -> Trigonometric Function5/1
  Trigonometric Function5/1 -> Gain5/1
  Math Function5/1 -> Add4/2
  Constant5/1 -> Math Function5/1
  Constant4/1 -> Math Function4/1
